simulink model "hc12_pwm"  (Simulink 6.0)
settings: Solver=FixedStepDiscrete  StartTime=0.0  StopTime=100000  FixedStep=hc12_base_st  RelTol=1e-3
PreLoadFcn:
  | [hc12_base_st] = hc12_closest_st(0.065536,16000000);
undefined symbols (not defined in the file or in its folder): hc12_base_st
libraries: hc12drivers x8
settings Model: Creator=The MathWorks Inc.  LastModifiedBy=batserve  ExtModeAutoUpdateStatusClock=off  ProdHWDeviceType=Motorola HC12
settings DataIOCC: SignalLoggingName=sigsOut
settings OptimizationCC: InlineParams=on  InlineInvariantSignals=off  ZeroExternalMemoryAtStartup=off  ZeroInternalMemoryAtStartup=off  OptimizeModelRefInitCode=on  LifeSpan=1
settings DebuggingCC: CheckExecutionContextPreStartOutputMsg=on  CheckExecutionContextRuntimeOutputMsg=on  SolverPrmCheckMsg=none
settings HardwareCC: ProdBitPerInt=16  ProdEndianess=BigEndian  ProdWordSize=16  ProdHWDeviceType=Motorola HC12
settings RTWCC: SystemTargetFile=hc12.tlc  TemplateMakefile=hc12_default_tmf  GenerateReport=on  RetainRTWFile=on  ProcessScript=hc12_make_rtw_hook  IncludeHyperlinkInReport=on  LaunchReport=on
settings CodeAppCC: IgnoreCustomStorageClasses=off
settings STFCustomTargetCC: TargetFcnLib=ansi_tfl_tmw.mat  GenFloatMathFcnCalls=ANSI_C  ModelReferenceCompliant=off  IncludeMdlTerminateFcn=off  CombineOutputUpdateFcns=on  SuppressErrorStatus=on  ERTCustomFileBanners=on  SupportAbsoluteTime=off  SupportNonFinite=off  SupportComplex=off  PurelyIntegerCode=on  SupportContinuousTime=off  SupportNonInlinedSFcns=off  SystemTargetFile=hc12.tlc
settings ERTTargetCC: TargetFcnLib=ansi_tfl_tmw.mat  GenFloatMathFcnCalls=ANSI_C  ModelReferenceCompliant=off  IncludeMdlTerminateFcn=off  SuppressErrorStatus=on  SupportAbsoluteTime=off  SupportNonFinite=off  SupportComplex=off  PurelyIntegerCode=on  RootIOFormat=Individual Arguments  ERTCustomFileTemplate=hc12_file_process.tlc  InitialValueSource=Model
settings CustomProperty: DataType=RTWOptions_EnumType__toolbox_rtw_targets_hc12_hc12_hc12_PWMPrescalerA  Value=1
settings EnumStrPairs: String=1

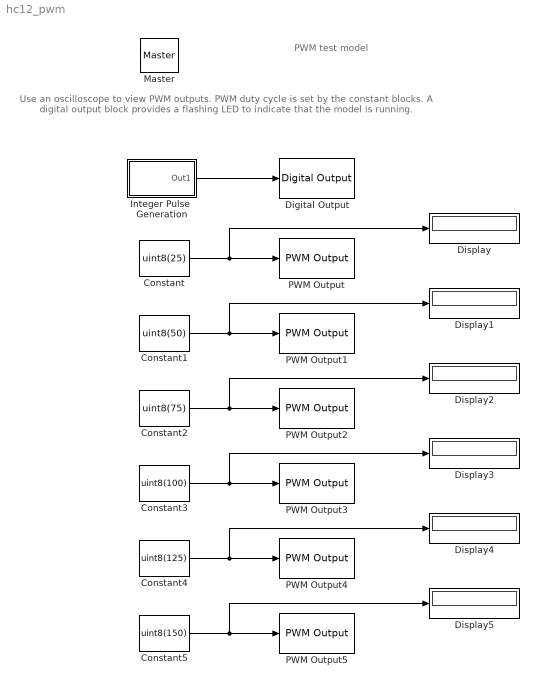
== system hc12_pwm ==
  note: PWM test model
  note: Use an oscilloscope to view PWM outputs. PWM
      | duty cycle is set by the constant blocks.
      |
      | A digital output block provides a flashing LED to
      | indicate that the model is running.
  Constant : Constant  Value=uint8(25)
  Constant1 : Constant  Value=uint8(50)
  Constant2 : Constant  Value=uint8(75)
  Constant3 : Constant  Value=uint8(100)
  Constant4 : Constant  Value=uint8(125)
  Constant5 : Constant  Value=uint8(150)
  Digital Output : hc12drivers/Digital Output  doport=B
  Display{,1..5} (6 alike) : Display
  Integer Pulse  Generation : Subsystem  PropExecContextAcrossSSBoundary=on
  Master : hc12drivers/Master  Tag=HardwareResourceMaster  Priority=100  osc=16000000  desiredST=hc12_base_st
  PWM Output : hc12drivers/PWM Output  channel=0  polaritybit=off  clkbit=off  caebit=off  pwmper=255
  PWM Output1 : hc12drivers/PWM Output  channel=1  polaritybit=off  clkbit=off  caebit=off  pwmper=255
  PWM Output2 : hc12drivers/PWM Output  channel=2  polaritybit=off  clkbit=off  caebit=off  pwmper=255
  PWM Output3 : hc12drivers/PWM Output  channel=3  polaritybit=off  clkbit=off  caebit=off  pwmper=255
  PWM Output4 : hc12drivers/PWM Output  channel=4  polaritybit=off  clkbit=off  caebit=off  pwmper=255
  PWM Output5 : hc12drivers/PWM Output  channel=5  polaritybit=off  clkbit=off  caebit=off  pwmper=255
  wires:
  Constant/1 -> Display/1, PWM Output/1
  Constant1/1 -> Display1/1, PWM Output1/1
  Constant2/1 -> Display2/1, PWM Output2/1
  Constant3/1 -> Display3/1, PWM Output3/1
  Constant4/1 -> Display4/1, PWM Output4/1
  Constant5/1 -> Display5/1, PWM Output5/1
  Integer Pulse  Generation/1(Out1) -> Digital Output/1

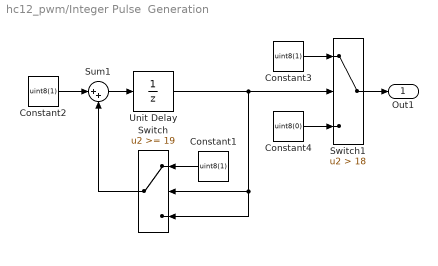
== system hc12_pwm/Integer Pulse  Generation ==
  Constant1 : Constant  Orientation=left  Value=uint8(1)
  Constant2 : Constant  Value=uint8(1)
  Constant3 : Constant  Value=uint8(1)
  Constant4 : Constant  Value=uint8(0)
  Sum1 : Sum  Inputs=|++  SaturateOnIntegerOverflow=on
  Switch : Switch  Orientation=left  Threshold=19  SaturateOnIntegerOverflow=on  InputSameDT=on
  Switch1 : Switch  Criteria=u2 > Threshold  Threshold=18  SaturateOnIntegerOverflow=on
  Unit Delay : UnitDelay  X0=uint8(0)  SampleTime=hc12_base_st
  Out1 : Outport
  wires:
  Switch1/1 -> Out1/1
  Constant4/1 -> Switch1/3
  Constant3/1 -> Switch1/1
  Switch/1 -> Sum1/2
  Constant2/1 -> Sum1/1
  Sum1/1 -> Unit Delay/1
  Constant1/1 -> Switch/1
  Unit Delay/1 -> Switch/3, Switch/2, Switch1/2
